simulink model "spwm_pulse_gen"  (R2023b)
settings: Solver=ode23t  StartTime=0.0  StopTime=0.1  MaxStep=1e-6  RelTol=1e-3
model workspace (MAT data in the model file):
  carrier_freq = 1
libraries: simulink x4
settings Model: Creator=ixale  LastModifiedBy=ixale

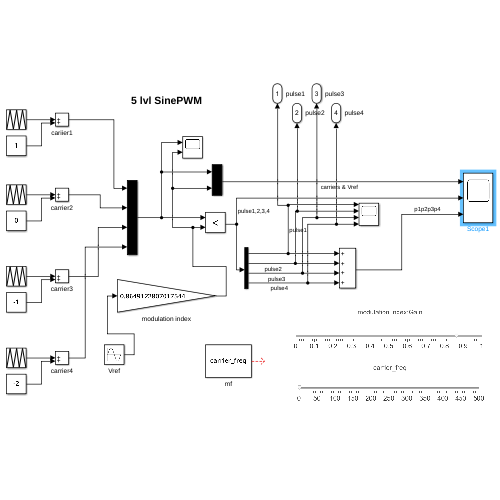
[thumbnail: Simulink's stored preview of the top-level diagram]
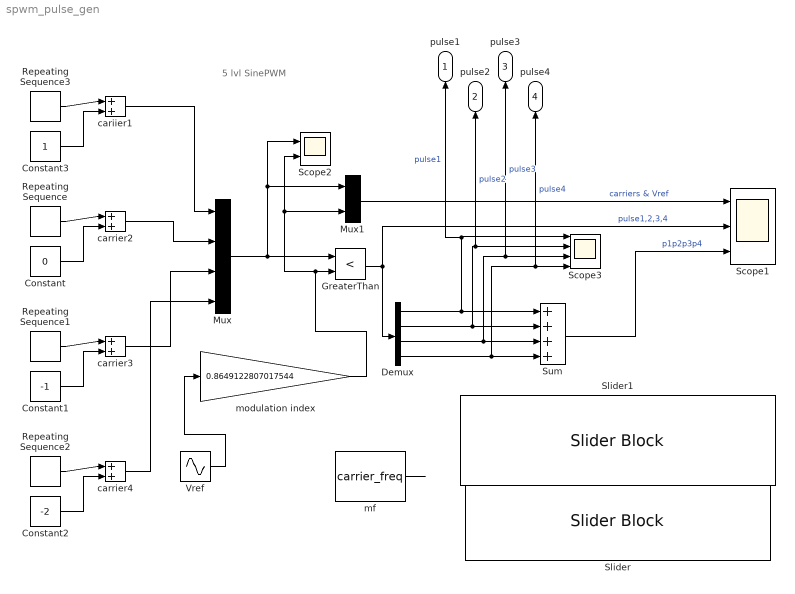
== system spwm_pulse_gen ==
  note: 5 lvl SinePWM
  Constant : Constant  Value=0
  Constant1 : Constant  Value=-1
  Constant2 : Constant  Value=-2
  Constant3 : Constant
  Demux : Demux
  GreaterThan : RelationalOperator  Operator=<  OutDataTypeStr=boolean  RndMeth=Simplest  InputSameDT=off
  Mux : Mux
  Mux1 : Mux  Inputs=2
  Repeating Sequence{,1..3} (4 alike) : simulink/Sources/Repeating Sequence  rep_seq_t=[0 0.5 1] / (50 * carrier_freq)  rep_seq_y=[0 1 0]
  Scope1 : Scope  NumInputPorts=3
  Scope2 : Scope  NumInputPorts=2
  Scope3 : Scope  NumInputPorts=4
  Slider : SliderBlock  ScaleMax=500
  Slider1 : SliderBlock  ScaleMax=1  TickInterval=0.1
  Sum : Sum  Inputs=++++
  Vref : Sin  Amplitude=2  Frequency=2*pi*50  SampleTime=0
  cariier1 : Sum  Inputs=|++
  carrier2 : Sum  Inputs=|++
  carrier3 : Sum  Inputs=|++
  carrier4 : Sum  Inputs=|++
  mf : Constant  Value=carrier_freq
  modulation index : Gain  Gain=0.8649122807017544
  pulse1 : Outport
  pulse2 : Outport  Port=2
  pulse3 : Outport  Port=3
  pulse4 : Outport  Port=4
  wires:
  Demux/3 -> pulse3/1, Scope3/3, Sum/3  "pulse3"
  Repeating Sequence3/1 -> cariier1/1
  carrier2/1 -> Mux/2
  Demux/1 -> pulse1/1, Scope3/1, Sum/1  "pulse1"
  Constant1/1 -> carrier3/2
  Repeating Sequence1/1 -> carrier3/1
  mf/1 -> ?
  Mux1/1 -> Scope1/1  "carriers & Vref"
  Vref/1 -> modulation index/1
  Sum/1 -> Scope1/3  "p1p2p3p4"
  GreaterThan/1 -> Scope1/2, Demux/1  "pulse1,2,3,4"
  modulation index/1 -> Mux1/2, Scope2/2, GreaterThan/2
  Demux/4 -> Sum/4, pulse4/1, Scope3/4  "pulse4"
  Constant3/1 -> cariier1/2
  Demux/2 -> Sum/2, pulse2/1, Scope3/2  "pulse2"
  Constant/1 -> carrier2/2
  Repeating Sequence2/1 -> carrier4/1
  carrier4/1 -> Mux/4
  cariier1/1 -> Mux/1
  Constant2/1 -> carrier4/2
  Mux/1 -> Scope2/1, Mux1/1, GreaterThan/1
  Repeating Sequence/1 -> carrier2/1
  carrier3/1 -> Mux/3
